simulink model "model2"  (R2024b)
settings: Solver=VariableStepAuto  StartTime=0.0  StopTime=1  MaxStep=1e-2  RelTol=1e-3
libraries: simulink x1
settings Model: Creator=mehmetcanevi  LastModifiedBy=mehmetcanevi

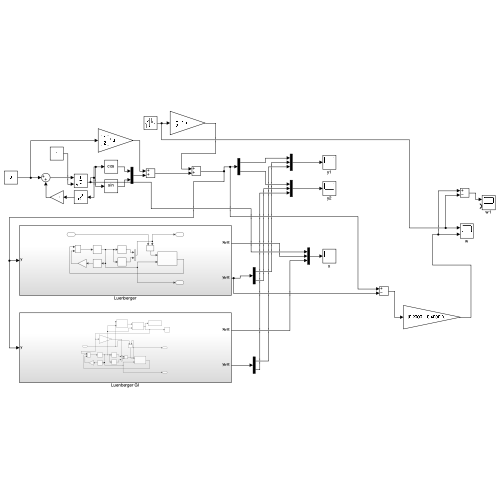
[thumbnail: Simulink's stored preview of the top-level diagram]
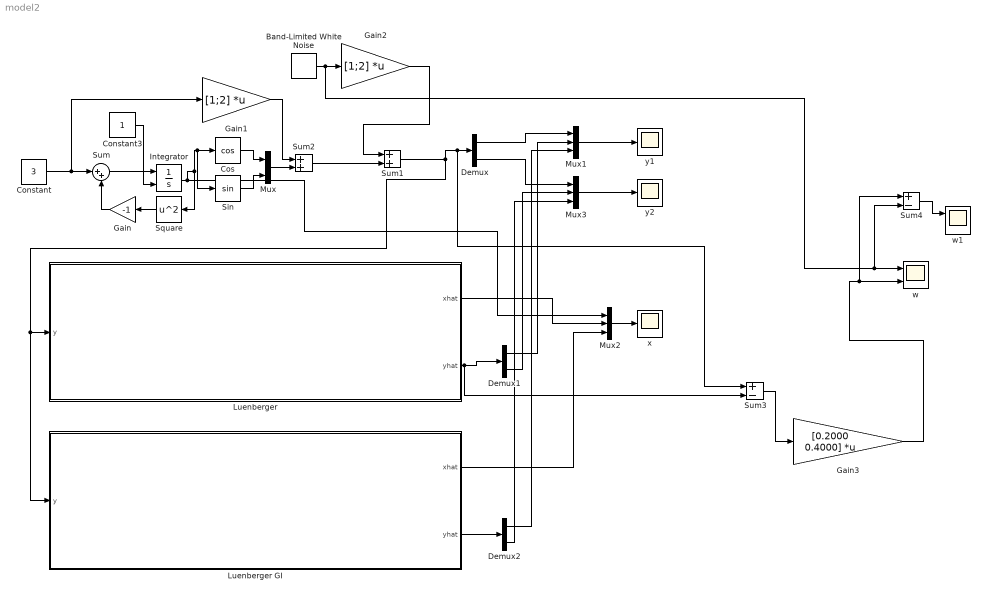
== system model2 ==
  Band-Limited White Noise : simulink/Sources/Band-Limited White Noise  Cov=[0.1]  Ts=0.01  seed=[23341]
  Constant : Constant  Value=3
  Constant3 : Constant
  Cos : Trigonometry  Operator=cos
  Demux : Demux  Outputs=2
  Demux1 : Demux  Outputs=2
  Demux2 : Demux  Outputs=2
  Gain : Gain  Gain=-1
  Gain1 : Gain  Gain=[1;2]  Multiplication=Matrix(K*u)
  Gain2 : Gain  Gain=[1;2]  Multiplication=Matrix(K*u)
  Gain3 : Gain  Gain="[0.2000    0.4000]"  Multiplication=Matrix(K*u)
  Integrator : Integrator  InitialConditionSource=external
  Luenberger : Subsystem
  Luenberger GI : Subsystem
  Mux : Mux  Inputs=2
  Mux1 : Mux  Inputs=3
  Mux2 : Mux  Inputs=3
  Mux3 : Mux  Inputs=3
  Sin : Trigonometry
  Square : Math  Operator=square
  Sum : Sum  Inputs=|++
  Sum1 : Sum
  Sum2 : Sum
  Sum3 : Sum  Inputs=+-
  Sum4 : Sum  Inputs=+-
  w : Scope  NumInputPorts=2
  w1 : Scope  NumInputPorts=2
  x : Scope
  y1 : Scope
  y2 : Scope
  wires:
  Integrator/1 -> Square/1, Sin/1, Cos/1, Mux2/1
  Sum/1 -> Integrator/1
  Cos/1 -> Mux/1
  Square/1 -> Gain/1
  Gain/1 -> Sum/2
  Constant3/1 -> Integrator/2
  Sin/1 -> Mux/2
  Mux/1 -> Sum2/2
  Constant/1 -> Sum/1, Gain1/1
  Gain1/1 -> Sum2/1
  Sum1/1 -> Sum3/1, Demux/1, Luenberger GI/1(y), Luenberger/1(y)
  Mux2/1 -> x/1
  Luenberger/1(xhat) -> Mux2/2
  Luenberger GI/1(xhat) -> Mux2/3
  Demux/1 -> Mux1/1
  Mux1/1 -> y1/1
  Mux3/1 -> y2/1
  Demux/2 -> Mux3/1
  Luenberger/2(yhat) -> Sum3/2, Demux1/1
  Demux1/1 -> Mux1/2
  Demux1/2 -> Mux3/2
  Luenberger GI/2(yhat) -> Demux2/1
  Demux2/1 -> Mux1/3
  Demux2/2 -> Mux3/3
  Sum2/1 -> Sum1/2
  Gain2/1 -> Sum1/1
  Sum3/1 -> Gain3/1
  Gain3/1 -> Sum4/1, w/2
  Sum4/1 -> w1/1
  Band-Limited White Noise/1 -> Sum4/2, w/1, Gain2/1

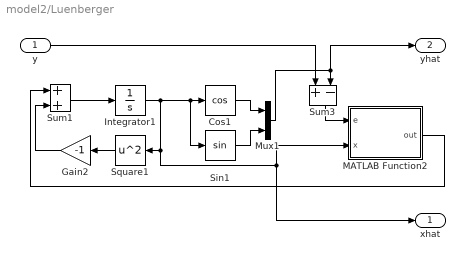
== system model2/Luenberger ==
  y : Inport
  Cos1 : Trigonometry  Operator=cos
  Gain2 : Gain  Gain=-1
  Integrator1 : Integrator
  MATLAB Function2 : MATLAB Function  TreatAsAtomicUnit=on
  Mux1 : Mux  Inputs=2
  Sin1 : Trigonometry
  Square1 : Math  Operator=square
  Sum1 : Sum
  Sum3 : Sum  Inputs=+-
  xhat : Outport
  yhat : Outport  Port=2
  wires:
  Sin1/1 -> Mux1/2
  Mux1/1 -> yhat/1, Sum3/2
  Integrator1/1 -> Sin1/1, Cos1/1, MATLAB Function2/2(x), xhat/1, Square1/1
  Cos1/1 -> Mux1/1
  Sum3/1 -> MATLAB Function2/1(e)
  MATLAB Function2/1(out) -> Sum1/1
  Square1/1 -> Gain2/1
  Sum1/1 -> Integrator1/1
  Gain2/1 -> Sum1/2
  y/1 -> Sum3/1

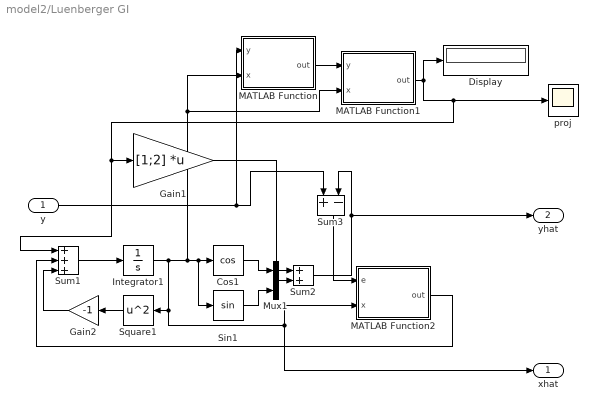
== system model2/Luenberger GI ==
  y : Inport
  Cos1 : Trigonometry  Operator=cos
  Display : Display
  Gain1 : Gain  Gain=[1;2]  Multiplication=Matrix(K*u)
  Gain2 : Gain  Gain=-1
  Integrator1 : Integrator
  MATLAB Function : MATLAB Function  TreatAsAtomicUnit=on
  MATLAB Function1 : MATLAB Function  TreatAsAtomicUnit=on
  MATLAB Function2 : MATLAB Function  TreatAsAtomicUnit=on
  Mux1 : Mux  Inputs=2
  Sin1 : Trigonometry
  Square1 : Math  Operator=square
  Sum1 : Sum  Inputs=+++
  Sum2 : Sum
  Sum3 : Sum  Inputs=+-
  proj : Scope
  xhat : Outport
  yhat : Outport  Port=2
  wires:
  Gain2/1 -> Sum1/3
  Sum1/1 -> Integrator1/1
  Square1/1 -> Gain2/1
  MATLAB Function2/1(out) -> Sum1/2
  Sum3/1 -> MATLAB Function2/1(e)
  Cos1/1 -> Mux1/1
  Integrator1/1 -> Square1/1, xhat/1, MATLAB Function2/2(x), MATLAB Function1/2(x), MATLAB Function/2(x), Cos1/1, Sin1/1
  Sum2/1 -> yhat/1, Sum3/2
  Sin1/1 -> Mux1/2
  MATLAB Function/1(out) -> MATLAB Function1/1(y)
  y/1 -> MATLAB Function/1(y), Sum3/1
  MATLAB Function1/1(out) -> Display/1, Sum1/1, Gain1/1, proj/1
  Mux1/1 -> Sum2/2
  Gain1/1 -> Sum2/1

== matlab function model2/Luenberger GI/MATLAB Function ==
  data: y input; out output; x input
function out= fcn(y,x)
out=[sin(x)^2, -sin(x)*cos(x);-sin(x)*cos(x), cos(x)^2]*y;
end

== matlab function model2/Luenberger/MATLAB Function2 ==
  data: e input; out output; x input
function out= fcn(e,x)
lambda=-10;
l2=(lambda+2*x-sin(x))/(-2*sin(x)-cos(x));
l1=1-2*l2;
out=[l1,l2]*e;
end

== matlab function model2/Luenberger GI/MATLAB Function2 ==
  data: e input; out output; x input
function out= fcn(e,x)
lambda=-10;
l2=(lambda+2*x-sin(x))/(-2*sin(x)-cos(x));
l1=1-2*l2;
out=[l1,l2]*e;
end

== matlab function model2/Luenberger GI/MATLAB Function1 ==
  data: y input; out output; x input
function out= fcn(y,x)
out=[-(sin(2*x) + cos(x)^2 - 1), cos(x)*(2*cos(x) - sin(x))]/(3*cos(x)^2 - 2*sin(2*x) + 1)*y;
end
